simulink model "sph_control_sim"  (Simulink 8.8)
settings: Solver=FixedStepDiscrete  StartTime=0.0  StopTime=20  RelTol=1e-3
InitFcn:
  | if exist('sph') && isvalid(sph) && sph.Status(1)=='o' && ping(sph),
  | [x0,y0]=readLocator(sph);
  | sph.BackLEDBrightness=100;
  | else
  | error('Make sure a valid and connected sphero variable named "sph" exist in the workspace before running this example');
  | end
undefined symbols (not defined in the file or in its folder): sfun3d, x0
undefined symbols (not defined in the file): y0
libraries: sphero_lib x4
settings Model: Creator=gcampa  LastModifiedBy=gcampa
settings DataIOCC: SignalLoggingSaveFormat=Dataset
settings OptimizationCC: BlockReduction=off  BooleanDataType=off
settings DebuggingCC: SaveWithParameterizedLinksMsg=none  SignalResolutionControl=TryResolveAllWithWarning  FcnCallInpInsideContextMsg=error  StateNameClashWarn=none
settings HardwareCC: TargetUnknown=on
settings GRTTargetCC: CombineOutputUpdateFcns=on  GRTInterface=off

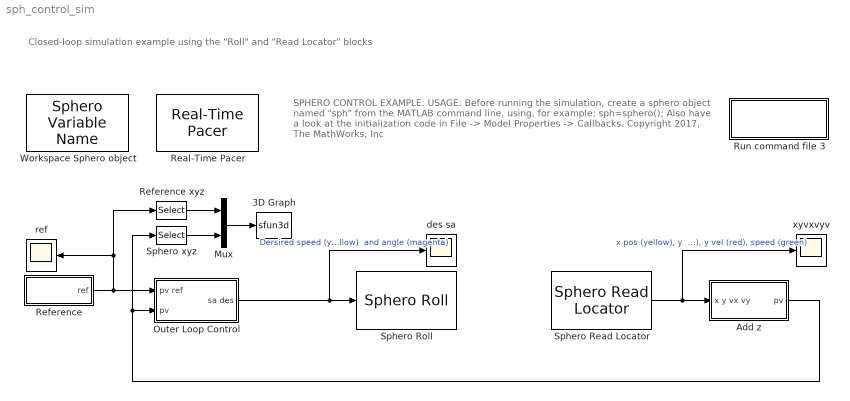
== system sph_control_sim ==
  note: SPHERO CONTROL EXAMPLE: USAGE:
      | Before running the simulation, create a sphero object named "sph" from the MATLAB
      | command line, using, for example: sph=sphero(); Also have a look at the initialization
      | code in File -> Model Properties -> Callbacks.     Copyright 2017, The MathWorks, Inc
  note: Closed-loop simulation example using the "Roll" and "Read Locator" blocks
  3D Graph : S-Function  LoadFcn=sfun3d([],[],[],'LoadBlock')  StartFcn=sfun3d([],[],[],'Start')  StopFcn=sfun3d([],[],[],'Stop')  FunctionName=sfun3d  Parameters=ax,T,np,cp,gd,ls,mk  SFunctionDeploymentMode=off  EnableBusSupport=off  mask(3D Graph){np=2, ax=[double(x0)-10 double(x0)+50 double(y0)-10 double(y0)+50  -10 10], cp=[10 10 20], gd=on, ls=-, mk=none, T=0.1}
      mask prompts: np "Number of point (lines)"; ax "[xmin xmax  ymin ymax zmin zmax]"; cp "Camera position (use [0 0 1] for 2D XY view)"; gd "Grid (on|off)"; ls "LineStyle"; mk "Marker"; T "Sampling Time"
      mask help:
      | This block plots the position of several points in the XYZ space. The input contains the coordinates of all the points (x1,y1,z1,x2,y2,z2,...).
      | The number of points (lines), the XYZ ranges, camera position, grid, linestyle, marker and sampling time, can be set as mask parameters.
      settings: CopyFcn=sfun3d([],[],[],'CopyBlock')  DeleteFcn=sfun3d([],[],[],'DeleteBlock')  NameChangeFcn=sfun3d([],[],[],'NameChange')
      mask Help:
      | This block plots the position of several points in the XYZ space. The input contains the coordinates of all the points (x1,y1,z1,x2,y2,z2,...).
      | The number of points (lines), the XYZ ranges, camera position, grid, linestyle, marker and sampling time, can be set as mask parameters.
      mask TypeOptions ls: - | -- | : | -. | none
      mask TypeOptions mk: none | . | + | o | * | x | square | diamond | v | ^ | > | < | pentagram | hexagram
      mask Display: plot([.05 .95 .95 .05 .05],[.45 .45 .95 .95 .45], 0.5+cos(0:0.1:2*pi)*0.3,0.7+sin(0:0.1:2*pi)*0.2)
  Add z : Subsystem
  Mux : Mux  Inputs=[3 3]
  Outer Loop Control : Subsystem  mask(Velocity Command Generator){Kp=1.64, Kv=0.01, T=0.1}
      mask prompts: Kp "Position Error Gain"; Kv "Velocity Error Gain"; T "Sample Time"
      mask help:
      | The first input is a reference position and velocity vector,
      |   the second one is a current position and velocity vector.
      |   The outputs are desired speed and angle.
      mask Help:
      | The first input is a reference position and velocity vector,
      |   the second one is a current position and velocity vector.
      |   The outputs are desired speed and angle.
  Real-Time Pacer : sphero_lib/Real-Time Pacer  simTimePerRealTime=1
  Reference : Subsystem  mask(Reference Path Generation){Px=double(x0)+[0  40  40  0   0], Py=double(y0)+[0  0  40  40  0], Ph=[4 4 4 4 4], Pt=[0 5 10 15 20], T=0.1}
      mask prompts: Px "X Positions"; Py "Y Positions"; Ph "H Positions"; Pt "Time"; T "Sample Time"
      mask help: This block generates a 3D trajectory. The output is a vector containing the position and velocity of a point that sequentially visits each X,Y,Z position at the corrisponding time. The velocity is constant between one visited point and the next.
      mask Help: This block generates a 3D trajectory. The output is a vector containing the position and velocity of a point that sequentially visits each X,Y,Z position at the corrisponding time. The velocity is constant between one visited point and the next.
  Reference xyz : Selector  InputPortWidth=6  IndexOptions=Index vector (dialog)  Indices=1:3  OutputSizes=1
  Run command file 3 : Subsystem
      settings: OpenFcn=sphero_lib
      mask Display: disp('Open Main\nSimulink Library')
  Sphero Read Locator : sphero_lib/Sphero Read Locator  SpheroVarNumber=Existing workspace Sphero variable #1  T=0.1
  Sphero Roll : sphero_lib/Sphero Roll  SpheroVarNumber=Existing workspace Sphero variable #1  T=0.1
  Sphero xyz : Selector  InputPortWidth=6  IndexOptions=Index vector (dialog)  Indices=1:3  OutputSizes=1
  Workspace Sphero object : sphero_lib/Sphero Variable Name  Priority=3  SpheroVarNumber=Existing workspace Sphero variable #1  workspaceVarName=sph
  des sa : Scope
  ref : Scope
  xyvxvyv : Scope
  wires:
  Reference/1(ref) -> Outer Loop Control/1(pv ref), Reference xyz/1, ref/1
  Outer Loop Control/1(sa des) -> des sa/1, Sphero Roll/1  "Dersired speed (yellow)  and angle (magenta)"
  Sphero Read Locator/1 -> xyvxvyv/1, Add z/1(x y vx vy)  "x pos (yellow), y  pos (magenta), x vel (cyan), y vel (red), speed (green)"
  Add z/1(pv) -> Sphero xyz/1, Outer Loop Control/2(pv)
  Mux/1 -> 3D Graph/1
  Sphero xyz/1 -> Mux/2
  Reference xyz/1 -> Mux/1

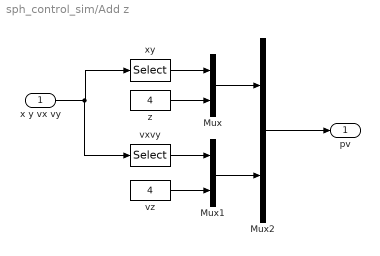
== system sph_control_sim/Add z ==
  x y vx vy : Inport
  Mux : Mux  Inputs=[2 1]
  Mux1 : Mux  Inputs=[2 1]
  Mux2 : Mux  Inputs=[3 3]
  vxvy : Selector  InputPortWidth=5  IndexOptions=Index vector (dialog)  Indices=3:4  OutputSizes=1
  vz : Constant  Value=4
  xy : Selector  InputPortWidth=5  IndexOptions=Index vector (dialog)  Indices=1:2  OutputSizes=1
  z : Constant  Value=4
  pv : Outport
  wires:
  x y vx vy/1 -> xy/1, vxvy/1
  Mux/1 -> Mux2/1
  vxvy/1 -> Mux1/1
  vz/1 -> Mux1/2
  Mux1/1 -> Mux2/2
  Mux2/1 -> pv/1
  z/1 -> Mux/2
  xy/1 -> Mux/1

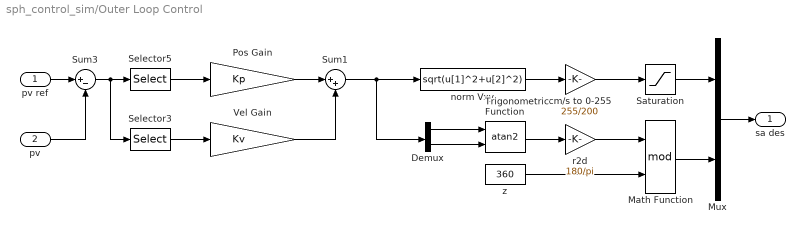
== system sph_control_sim/Outer Loop Control ==
  pv ref : Inport
  pv : Inport  Port=2
  Demux : Demux  Outputs=[1 1]
  Math Function : Math  Operator=mod  SaturateOnIntegerOverflow=on
  Mux : Mux  Inputs=[1 1]
  Pos Gain : Gain  Gain=Kp  SampleTime=T  SaturateOnIntegerOverflow=on  OutDataTypeStr=Inherit: Same as input  ParamDataTypeStr=Inherit: Same as input
  Saturation : Saturate  UpperLimit=255  LowerLimit=0
  Selector3 : Selector  InputPortWidth=6  IndexOptions=Index vector (dialog)  Indices=4:5  OutputSizes=1
  Selector5 : Selector  InputPortWidth=6  IndexOptions=Index vector (dialog)  Indices=1:2  OutputSizes=1
  Sum1 : Sum  Inputs=|++  SaturateOnIntegerOverflow=on  InputSameDT=on  OutDataTypeStr=Inherit: Same as first input
  Sum3 : Sum  Inputs=|+-  SaturateOnIntegerOverflow=on  InputSameDT=on  OutDataTypeStr=Inherit: Same as first input
  Trigonometric Function : Trigonometry  Operator=atan2
  Vel Gain : Gain  Gain=Kv  SampleTime=T  SaturateOnIntegerOverflow=on  OutDataTypeStr=Inherit: Same as input  ParamDataTypeStr=Inherit: Same as input
  cm/s to 0-255 : Gain  Gain=255/200  SaturateOnIntegerOverflow=on  OutDataTypeStr=Inherit: Same as input  ParamDataTypeStr=Inherit: Same as input
  norm Vxy : Fcn  Expr=sqrt(u[1]^2+u[2]^2)
  r2d : Gain  Gain=180/pi  SaturateOnIntegerOverflow=on  OutDataTypeStr=Inherit: Same as input  ParamDataTypeStr=Inherit: Same as input
  z : Constant  Value=360
  sa des : Outport
  wires:
  Demux/2 -> Trigonometric Function/2
  Demux/1 -> Trigonometric Function/1
  cm/s to 0-255/1 -> Saturation/1
  Saturation/1 -> Mux/1
  Mux/1 -> sa des/1
  norm Vxy/1 -> cm/s to 0-255/1
  Trigonometric Function/1 -> r2d/1
  Sum1/1 -> norm Vxy/1, Demux/1
  pv/1 -> Sum3/2
  pv ref/1 -> Sum3/1
  Selector5/1 -> Pos Gain/1
  Sum3/1 -> Selector5/1, Selector3/1
  Selector3/1 -> Vel Gain/1
  Vel Gain/1 -> Sum1/2
  Pos Gain/1 -> Sum1/1
  r2d/1 -> Math Function/1
  z/1 -> Math Function/2
  Math Function/1 -> Mux/2

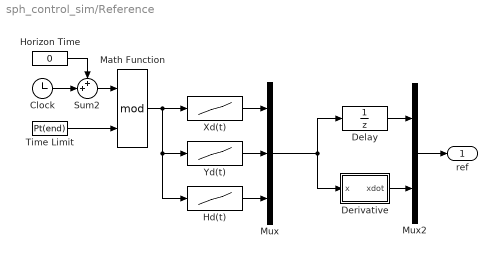
== system sph_control_sim/Reference ==
  Clock : Clock
  Delay : UnitDelay  InitialCondition=[Px(1) Py(1) Ph(1)]  SampleTime=T
  Derivative : Subsystem  mask(Time Derivative){x0=[Px(1) Py(1) Ph(1)]'-[Px(2)-Px(1) Py(2)-Py(1) Ph(2)-Ph(1)]'/(Pt(2)-Pt(1))*T, T=T}
      mask prompts: x0 "Initial Condition"; T "Sampling Time"
      mask help:
      | First order approximation of the time derivative of the input signal,
      |   the original one is buggy.
  Hd(t) : Lookup  InputValues=Pt  Table=Ph  SaturateOnIntegerOverflow=on
  Horizon Time : Constant  Value=0
  Math Function : Math  Operator=mod  SaturateOnIntegerOverflow=on
  Mux : Mux  Inputs=3
  Mux2 : Mux  Inputs=[3 3]
  Sum2 : Sum  Inputs=++|  SaturateOnIntegerOverflow=on  InputSameDT=on  OutDataTypeStr=Inherit: Same as first input
  Time Limit : Constant  Value=Pt(end)
  Xd(t) : Lookup  InputValues=Pt  Table=Px  SaturateOnIntegerOverflow=on
  Yd(t) : Lookup  InputValues=Pt  Table=Py  SaturateOnIntegerOverflow=on
  ref : Outport
  wires:
  Mux2/1 -> ref/1
  Derivative/1(xdot) -> Mux2/2
  Delay/1 -> Mux2/1
  Xd(t)/1 -> Mux/1
  Yd(t)/1 -> Mux/2
  Hd(t)/1 -> Mux/3
  Sum2/1 -> Math Function/1
  Horizon Time/1 -> Sum2/1
  Clock/1 -> Sum2/2
  Math Function/1 -> Xd(t)/1, Yd(t)/1, Hd(t)/1
  Time Limit/1 -> Math Function/2
  Mux/1 -> Delay/1, Derivative/1(x)

== system sph_control_sim/Run command file 3 ==

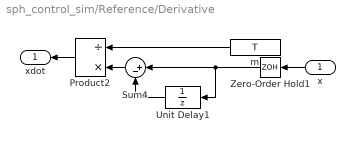
== system sph_control_sim/Reference/Derivative ==
  x : Inport
  Product2 : Product  Inputs=/*  SaturateOnIntegerOverflow=on  RndMeth=Zero  InputSameDT=on  OutDataTypeStr=Inherit: Same as first input
  Sum4 : Sum  Inputs=|+-  SaturateOnIntegerOverflow=on  InputSameDT=on  OutDataTypeStr=Inherit: Same as first input
  Unit Delay1 : UnitDelay  InitialCondition=x0  SampleTime=T
  Zero-Order Hold1 : ZeroOrderHold  SampleTime=T
  m : Constant  Value=T
  xdot : Outport
  wires:
  x/1 -> Zero-Order Hold1/1
  Product2/1 -> xdot/1
  m/1 -> Product2/1
  Zero-Order Hold1/1 -> Unit Delay1/1, Sum4/1
  Unit Delay1/1 -> Sum4/2
  Sum4/1 -> Product2/2
